simulink model "interpolation_nD_TestGen26"  (R2017b)
settings: Solver=FixedStepDiscrete  StartTime=0.0  StopTime=10.0  RelTol=1e-3
settings Model: Creator=ktrinh  LastModifiedBy=ktrinh
settings DebuggingCC: ParameterOverflowMsg=none

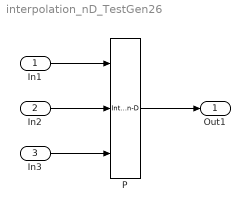
== system interpolation_nD_TestGen26 ==
  In1 : Inport  OutMin=0  OutMax=2  OutDataTypeStr=Bus: kfBus  PortDimensions=3  BusOutputAsStruct=on
  In2 : Inport  Port=2  OutMin=0  OutMax=5
  In3 : Inport  Port=3  PortDimensions=[2 5]
  P : Interpolation_n-D  InitFcn=|  TableSource=Input port  InterpMethod=Nearest  RequireIndexFractionAsBus=on  NumSelectionDims=1  OutDataTypeStr=int16  InternalRulePriority=Speed  RndMeth=Simplest  IntermediateResultsDataTypeStr=int8
      | elems(1) = Simulink.BusElement;
      | elems(1).Name = 'Index';
      | elems(1).DataType = 'int8';
      | elems(2) = Simulink.BusElement;
      | elems(2).Name = 'Fraction';
      | elems(2).DataType = 'double';
      | kfBus = Simulink.Bus;
      | kfBus.Elements = elems;
      | clear elems;
      | assignin('base', 'kfBus', kfBus);
      settings: InputPortMap=u0,u1,p2
  Out1 : Outport
  wires:
  In1/1 -> P/1
  In2/1 -> P/2
  In3/1 -> P/3
  P/1 -> Out1/1
